simulink library "adrc_lib"  (R2018b)
settings: Solver=VariableStepAuto  StartTime=0.0  StopTime=10.0  RelTol=1e-3
settings Model: Creator=zouji  LastModifiedBy=zouji

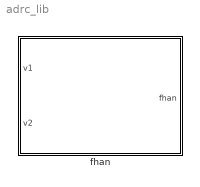
== system adrc_lib ==
  fhan : Subsystem  mask{r0=0, h0=0}
      mask DialogControl ParameterGroupVar Prompt: fhan(v1,v2,r0,h0)

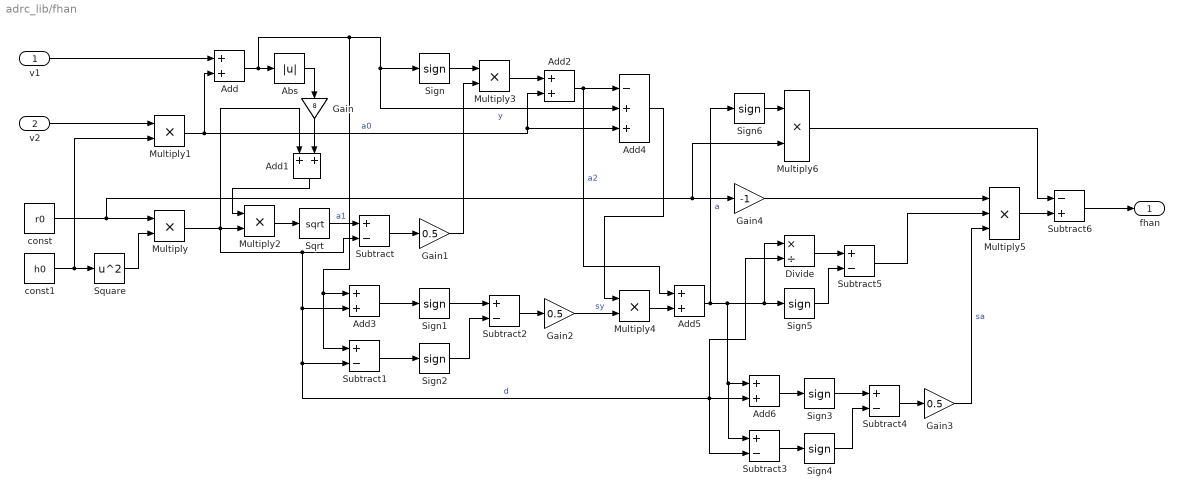
== system adrc_lib/fhan ==
  v1 : Inport
  v2 : Inport  Port=2
  Abs : Abs
  Add{,1..3,5..6} (6 alike) : Sum  OutDataTypeStr=Inherit: Same as first input
  Add4 : Sum  Inputs=-++
  Divide : Product  Inputs=*/
  Gain : Gain  Gain=8
  Gain1 : Gain  Gain=0.5  OutDataTypeStr=Inherit: Same as input
  Gain2 : Gain  Gain=0.5  OutDataTypeStr=Inherit: Same as input
  Gain3 : Gain  Gain=0.5  OutDataTypeStr=Inherit: Same as input
  Gain4 : Gain  Gain=-1  OutDataTypeStr=Inherit: Same as input
  Multiply{,1..3} (4 alike) : Product  OutDataTypeStr=Inherit: Same as first input
  Multiply4 : Product  OutDataTypeStr=single
  Multiply5 : Product  Inputs=3
  Multiply6 : Product  OutDataTypeStr=single
  Sign{,1..6} (7 alike) : Signum
  Sqrt : Sqrt  SaturateOnIntegerOverflow=on
  Square : Math  Operator=square  SaturateOnIntegerOverflow=on
  Subtract{,1..5} (6 alike) : Sum  Inputs=+-  OutDataTypeStr=Inherit: Same as first input
  Subtract6 : Sum  Inputs=-+  OutDataTypeStr=Inherit: Same as first input
  const : Constant  Value=r0  OutDataTypeStr=single
  const1 : Constant  Value=h0  OutDataTypeStr=single
  fhan : Outport
  wires:
  Sign1/1 -> Subtract2/1
  Add/1 -> Subtract1/1, Add3/1, Add4/2, Sign/1, Abs/1  "y"
  Multiply6/1 -> Subtract6/1
  Subtract4/1 -> Gain3/1
  Subtract3/1 -> Sign4/1
  Add6/1 -> Sign3/1
  Multiply/1 -> Subtract/2, Divide/2, Subtract3/2, Add6/2, Subtract1/2, Add3/2, Add1/1, Multiply2/2  "d"
  Add2/1 -> Add4/1, Add5/1  "a2"
  Add3/1 -> Sign1/1
  Gain3/1 -> Multiply5/3  "sa"
  Gain1/1 -> Multiply3/2
  Add1/1 -> Multiply2/1
  Sign6/1 -> Multiply6/1
  Multiply5/1 -> Subtract6/2
  Subtract5/1 -> Multiply5/2
  Sign3/1 -> Subtract4/1
  Square/1 -> Multiply/2
  Gain4/1 -> Multiply5/1
  Subtract2/1 -> Gain2/1
  Add5/1 -> Sign6/1, Sign5/1, Divide/1, Subtract3/1, Add6/1  "a"
  Multiply4/1 -> Add5/2
  Multiply1/1 -> Add4/3, Add2/2, Add/2  "a0"
  Abs/1 -> Gain/1
  Sqrt/1 -> Subtract/1  "a1"
  const/1 -> Multiply6/2, Gain4/1, Multiply/1
  v1/1 -> Add/1
  Divide/1 -> Subtract5/1
  Multiply3/1 -> Add2/1
  Add4/1 -> Multiply4/1
  Gain/1 -> Add1/2
  v2/1 -> Multiply1/1
  Subtract6/1 -> fhan/1
  Sign2/1 -> Subtract2/2
  Sign/1 -> Multiply3/1
  const1/1 -> Multiply1/2, Square/1
  Sign5/1 -> Subtract5/2
  Subtract/1 -> Gain1/1
  Sign4/1 -> Subtract4/2
  Gain2/1 -> Multiply4/2  "sy"
  Subtract1/1 -> Sign2/1
  Multiply2/1 -> Sqrt/1
